simulink model "PIDFInAL"  (R2022b)
settings: Solver=VariableStepAuto  StartTime=0.0  StopTime=240  RelTol=1e-3
values from neighbouring files (symbols this model uses):
  eul0 = [0; 0; 0]    [initialS.m]
  Irw = 5.7e-5*eye(3)    [initialS.m]
  Iw = 5.7e-5    (= 5.7e-05)    [initialS.m]
  Jt = [0.185 0 0; 0 0.144 0; 0 0 0.061]    [initialS.m]
  omega0 = [0; 0; 0]    [initialS.m]
  Q = [0; 0; 0; 0]    [initialS.m]
libraries: slpidlib x1
settings Model: Creator=Egraweb  LastModifiedBy=Egraweb
settings DebuggingCC: UnconnectedInputMsg=warning  UnconnectedOutputMsg=warning  UnconnectedLineMsg=warning
settings ModelReferenceCC: EnableRefExpFcnMdlSchedulingChecks=on
settings RTWCC: DLArmComputeVersion=19.05

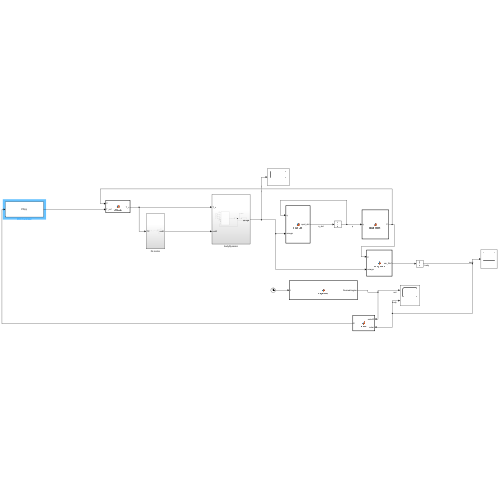
[thumbnail: Simulink's stored preview of the top-level diagram]
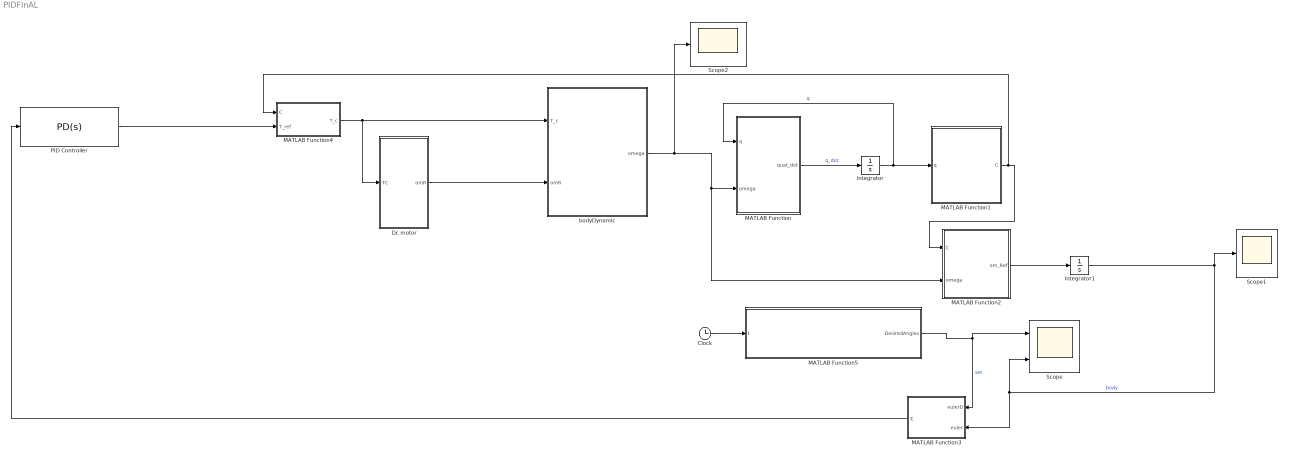
== system PIDFInAL ==
  Clock : Clock
  Dc motor : Subsystem
  Integrator : Integrator  InitialCondition=Q
  Integrator1 : Integrator  InitialCondition=eul0
  MATLAB Function : MATLAB Function  TreatAsAtomicUnit=on
  MATLAB Function1 : MATLAB Function  TreatAsAtomicUnit=on
  MATLAB Function2 : MATLAB Function  TreatAsAtomicUnit=on
  MATLAB Function3 : MATLAB Function  TreatAsAtomicUnit=on
  MATLAB Function4 : MATLAB Function  TreatAsAtomicUnit=on
  MATLAB Function5 : MATLAB Function  TreatAsAtomicUnit=on
  PID Controller : slpidlib/PID Controller  Controller=PD  Form=Parallel  TimeDomain=Continuous-time  UseExternalTs=off  SampleTime=-1  IntegratorMethod=Forward Euler  FilterMethod=Forward Euler  ControllerParametersSource=internal  P=1  I=1  UseKiTs=off  D=5  N=100  UseFilter=on  TunerSelectOption=Transfer Function Based (PID Tuner App)  InitialConditionSource=internal  InitialConditionForIntegrator=0  InitialConditionForFilter=0  DifferentiatorICPrevScaledInput=0  ExternalReset=none  TrackingMode=off  Kt=1  LimitOutput=off  SatLimitsSource=internal  UpperSaturationLimit=inf  LowerSaturationLimit=-inf  LinearizeAsGain=on  AntiWindupMode=none  Kb=1  LimitIntegrator=off  UpperIntegratorSaturationLimit=inf  LowerIntegratorSaturationLimit=-inf  POutMin=[]  POutMax=[]  IOutMin=[]  IOutMax=[]  DOutMin=[]  DOutMax=[]  NOutMin=[]  NOutMax=[]  SumOutMin=[]  SumOutMax=[]  SaturationOutMin=[]  SaturationOutMax=[]  PParamMin=[]  PParamMax=[]  IParamMin=[]  IParamMax=[]  DParamMin=[]  DParamMax=[]  NParamMin=[]  NParamMax=[]  KbParamMin=[]  KbParamMax=[]  KtParamMin=[]  KtParamMax=[]  KbOutMin=[]  KbOutMax=[]  KtOutMin=[]  KtOutMax=[]  IntegratorOutMin=[]  IntegratorOutMax=[]  FilterOutMin=[]  FilterOutMax=[]  SumI1OutMin=[]  SumI1OutMax=[]  SumI2OutMin=[]  SumI2OutMax=[]  SumI3OutMin=[]  SumI3OutMax=[]  SumI4OutMin=[]  SumI4OutMax=[]  SumDOutMin=[]  SumDOutMax=[]  DifferentiatorOutMin=[]  DifferentiatorOutMax=[]  FilterDiffOutCoefMin=[]  FilterDiffOutCoefMax=[]  ReciprocalOutMin=[]  ReciprocalOutMax=[]  SumDenOutMin=[]  SumDenOutMax=[]  SumNumOutMin=[]  SumNumOutMax=[]  DivideOutMin=[]  DivideOutMax=[]  UdiffTsProdOutMin=[]  UdiffTsProdOutMax=[]  NTsProdOutMin=[]  NTsProdOutMax=[]  UintegralTsProdOutMin=[]  UintegralTsProdOutMax=[]  UngainTsProdOutMin=[]  UngainTsProdOutMax=[]  ClampingZeroOutDataTypeStr=Inherit: Inherit via back propagation  ClampingZeroOutMin=[]  ClampingZeroOutMax=[]  FilterDenConstantOutDataTypeStr=Inherit: Inherit via back propagation  FilterDenConstantOutMin=[]  FilterDenConstantOutMax=[]  PCopyOutDataTypeStr=Inherit: Inherit via back propagation  PCopyOutMin=[]  PCopyOutMax=[]  NCopyOutDataTypeStr=Inherit: Inherit via back propagation  NCopyOutMin=[]  NCopyOutMax=[]  IntegratorContinuousStateAttributes=''  IntegratorStateMustResolveToSignalObject=off  IntegratorRTWStateStorageClass=Auto  FilterContinuousStateAttributes=''  FilterStateMustResolveToSignalObject=off  FilterRTWStateStorageClass=Auto  ParallelPVariant=InternalParameters  IdealPVariant=Disabled  IVariant=Disabled  DVariant=InternalParameters  IntegratorVariant=Disabled  SatVariant=Disabled  AWVariant=Disabled  PCopyVariant=Disabled  TRVariant=Disabled  FdbkBlocksVariant=Forward  IdealPFdbkVariant=Disabled  SatFdbkVariant=Disabled  DerivativeFilterVariant=ContFilter  NVariant=InternalParameters  NCopyVariant=Disabled  FilterICVariant=InternalICsFilter  IntegratorICVariant=Disabled  ExternalResetVariant=Disabled  TRSumVariant=Passthrough  SumFdbkVariant=Disabled  SumVariant=Sum_PD  TsampFilterVariant=InternalTs  TsampNgainVariant=Passthrough  TsampIntegralVariant=Disabled_SignalSpec  ExternalSaturationOutDataTypeStr=Inherit: Same as second input
  Scope : Scope  NumInputPorts=2
  Scope1 : Scope
  Scope2 : Scope
  bodyDynamic : Subsystem
  wires:
  MATLAB Function4/1(T_c) -> Dc motor/1(TC), bodyDynamic/1(T_c)
  MATLAB Function2/1(om_Ref) -> Integrator1/1
  Clock/1 -> MATLAB Function5/1(t)
  MATLAB Function5/1(DesiredAngles) -> Scope/1, MATLAB Function3/1(eulerD)  "set"
  Dc motor/1(omR) -> bodyDynamic/2(omR)
  bodyDynamic/1(omega) -> Scope2/1, MATLAB Function2/2(omega), MATLAB Function/2(omega)
  MATLAB Function1/1(C) -> MATLAB Function4/1(C), MATLAB Function2/1(C)
  MATLAB Function/1(quat_dot) -> Integrator/1  "q_dot"
  Integrator/1 -> MATLAB Function/1(q), MATLAB Function1/1(q)  "q"
  Integrator1/1 -> Scope1/1, Scope/2, MATLAB Function3/2(euler)  "body"
  PID Controller/1 -> MATLAB Function4/2(T_ref)
  MATLAB Function3/1(E) -> PID Controller/1

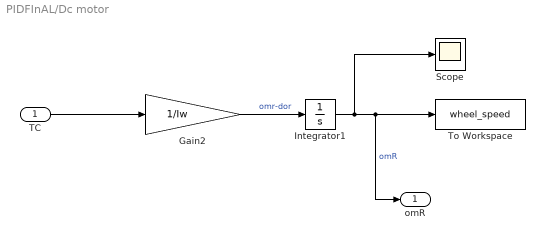
== system PIDFInAL/Dc motor ==
  TC : Inport
  Gain2 : Gain  Gain=1/Iw
  Integrator1 : Integrator  InitialCondition=[0;0;0]
  Scope : Scope
  To Workspace : ToWorkspace  VariableName=wheel_speed  SaveFormat=Timeseries  SampleTime=-1
  omR : Outport
  wires:
  Gain2/1 -> Integrator1/1  "omr-dor"
  Integrator1/1 -> Scope/1, omR/1, To Workspace/1  "omR"
  TC/1 -> Gain2/1

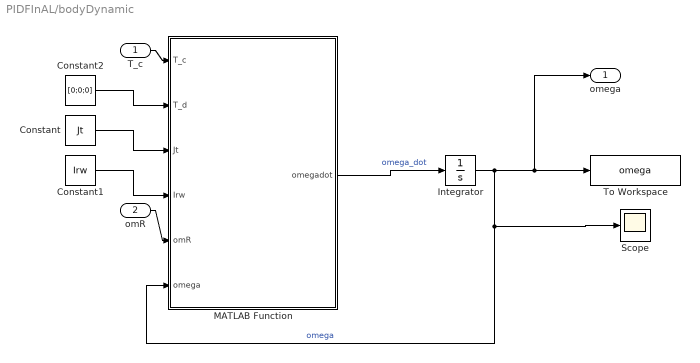
== system PIDFInAL/bodyDynamic ==
  T_c : Inport
  omR : Inport  Port=2
  Constant : Constant  Value=Jt
  Constant1 : Constant  Value=Irw
  Constant2 : Constant  Value=[0;0;0]
  Integrator : Integrator  InitialCondition=omega0
  MATLAB Function : MATLAB Function  TreatAsAtomicUnit=on
  Scope : Scope
  To Workspace : ToWorkspace  VariableName=omega  SaveFormat=Timeseries  SampleTime=-1
  omega : Outport
  wires:
  Integrator/1 -> omega/1, To Workspace/1, Scope/1, MATLAB Function/6(omega)  "omega"
  Constant/1 -> MATLAB Function/3(Jt)
  MATLAB Function/1(omegadot) -> Integrator/1  "omega_dot"
  T_c/1 -> MATLAB Function/1(T_c)
  omR/1 -> MATLAB Function/5(omR)
  Constant1/1 -> MATLAB Function/4(Irw)
  Constant2/1 -> MATLAB Function/2(T_d)

== matlab function PIDFInAL/MATLAB Function ==
  data: q input; quat_dot output; omega input
function quat_dot = quatDot(q,omega)


quat_dot=0.5*([0 -omega(1) -omega(2) -omega(3); omega(1) 0 omega(3) -omega(2); omega(2) -omega(3) 0 omega(1); omega(3) omega(2) -omega(1) 0])*q;

== matlab function PIDFInAL/bodyDynamic/MATLAB Function ==
  data: T_c input; T_d input; omegadot output; Jt input; Irw input; omR input; omega input
function omegadot = MotionEquation(T_c,T_d,Jt,Irw,omR,omega)

omegaS=[0 -omega(3) omega(2);
    omega(3) 0 -omega(1);
    -omega(2) omega(1) 0];
omegadot=Jt\(T_d+T_c-(omegaS)*(Jt*omega+Irw*omR));

== matlab function PIDFInAL/MATLAB Function1 ==
  data: q input; C output
function C = quat2rotm (q)



C = [1 - 2*(q(3)^2 + q(4)^2),   2*(q(2)*q(3) - q(1)*q(4)),       2*(q(2)*q(4) + q(1)*q(3));
     2*(q(2)*q(3) + q(1)*q(4)),   1 - 2*(q(2)^2 + q(4)^2),         2*(q(3)*q(4) - q(1)*q(2));
     2*(q(2)*q(4) - q(1)*q(2)),       2*(q(3)*q(4) + q(1)*q(2)) ,  1 - 2*(q(2)^2 + q(3)^2)];

== matlab function PIDFInAL/MATLAB Function2 ==
  data: C input; om_Ref output; omega input
function om_Ref = Body2Ref(C , omega)

om_Ref = C * omega;

== matlab function PIDFInAL/MATLAB Function3 ==
  data: eulerD input; E output; euler input
function E = error(eulerD , euler)

E = eulerD - euler;

== matlab function PIDFInAL/MATLAB Function4 ==
  data: C input; T_ref input; T_c output
function T_c = ref2body(C ,T_ref)

T_c = transpose(C)* T_ref;

== matlab function PIDFInAL/MATLAB Function5 ==
  data: t input; DesiredAngles output
function DesiredAngles = trajectory(t)
roll  = 0;
pitch = 2;
yaw   = 2;
eulerD = [roll; pitch; yaw];
DesiredAngles = eulerD;
